simulink subsystem "s0518_switching_policy3"  (R2019b)
settings: Solver=VariableStepAuto  StartTime=0.0  StopTime=10.0  RelTol=1e-3
undefined symbols (not defined in the file): __PRM__SERIALIZED__DATA__, SubsystemReferenceBlock
settings Model: Creator=paolo  LastModifiedBy=giaco

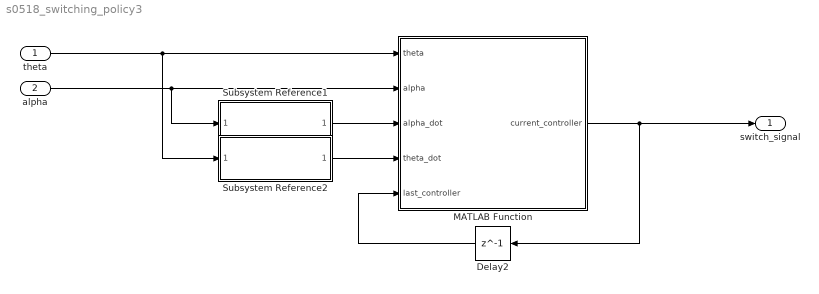
== system s0518_switching_policy3 ==
  theta : Inport
  alpha : Inport  Port=2
  Delay2 : Delay  DelayLength=1  InitialCondition=3
  MATLAB Function : MATLAB Function  TreatAsAtomicUnit=on
  Subsystem Reference1 : Subsystem  BlockKeywords=__PRM__SERIALIZED__DATA__:SubsystemReferenceBlock  ReferencedSubsystem=Filtered_Derivative  num=num_der_filter  den=den_der_filter
  Subsystem Reference2 : Subsystem  BlockKeywords=__PRM__SERIALIZED__DATA__:SubsystemReferenceBlock  ReferencedSubsystem=Filtered_Derivative  num=num_der_filter  den=den_der_filter
  switch_signal : Outport
  wires:
  theta/1 -> MATLAB Function/1(theta), Subsystem Reference2/1
  alpha/1 -> Subsystem Reference1/1, MATLAB Function/2(alpha)
  MATLAB Function/1(current_controller) -> Delay2/1, switch_signal/1
  Delay2/1 -> MATLAB Function/5(last_controller)
  Subsystem Reference1/1 -> MATLAB Function/3(alpha_dot)
  Subsystem Reference2/1 -> MATLAB Function/4(theta_dot)

== matlab function s0518_switching_policy3/MATLAB Function ==
  data: theta input; current_controller output; alpha input; alpha_dot input; theta_dot input; last_controller input double
function current_controller = PP_enabler(theta, alpha, alpha_dot, theta_dot, last_controller)
 
% current_controller = 1 for swing up, 2 for PP up, 3 for PP down, 4 for
% free falling

alpha_diff = alpha*180/pi - 180;
theta = theta*180/pi;
 
stop_condition = false;
while ~stop_condition
    if alpha_diff > 180
        alpha_diff = alpha_diff - 360;
    elseif alpha_diff < -180
        alpha_diff = alpha_diff + 360;
    else
        stop_condition = true;
    end
end
 
if last_controller == 1 && (abs(alpha_diff) < 30 && abs(alpha_dot) < 5 && abs(theta) < 120)
    current_controller = 2;
elseif last_controller == 2 && (abs(alpha_diff) > 50 || abs(theta) > 125) 
    current_controller = 4;
elseif last_controller == 3 && (abs(alpha_diff) > 178 && abs(theta) < 2 && abs(alpha_dot) < 0.5 && abs(theta_dot) < 0.5) 
    current_controller = 1;
elseif last_controller == 4 && (abs(alpha_diff) > 170 && abs(alpha_dot) < 22) 
    current_controller = 3;
else 
    current_controller = last_controller;
end
 
end
